simulink model "Smart_City_Communication_Infrastructure"  (R2024b)
settings: Solver=ode1  StartTime=0.0  StopTime=inf  FixedStep=Controller_Sample_Time  RelTol=1e-3  EnableMultiTasking=on
undefined symbols (not defined in the file or in its folder): DiscIntNeverNeededParam, qc_get_step_size
libraries: quarc_library x26, simulink x2
settings Model: SimulationMode=external  ExtModeTrigDuration=10000  Creator=PK  LastModifiedBy=user
settings SolverCC: AlgebraicLoopSolver=TrustRegion  PositivePriorityOrder=on
settings DataIOCC: ReturnWorkspaceOutputs=off
settings DebuggingCC: UnconnectedInputMsg=warning  UnconnectedOutputMsg=warning  UnconnectedLineMsg=warning  ArithmeticOperatorsInVariantConditions=warning
settings ModelReferenceCC: EnableRefExpFcnMdlSchedulingChecks=on
settings SFSimCC: SimUseLocalCustomCode=off  CustomCodeUndefinedFunction=UseInterfaceOnly
settings RTWCC: Description=QUARC Win64 Target Using Toolchain  SystemTargetFile=quarc_win64.tlc  TemplateMakefile=quarc_default_tmf  RTWUseLocalCustomCode=off  Toolchain=QUARC win64 | nmake (64-bit Windows)  BuildConfiguration=Faster Runs  GPUComputeCapability=3.5
settings CodeAppCC: StateflowObjectComments=on
settings STFCustomTargetCC: TargetLangStandard=C99 (ISO)  ConcurrentExecutionCompliant=on  GRTInterface=on  UseToolchainInfoCompliant=on  SystemTargetFile=quarc_win64.tlc
settings GRTTargetCC: ParMdlRefBuildCompliant=off  CompOptLevelCompliant=off  CombineOutputUpdateFcns=off  MatFileLogging=off  CPPClassGenCompliant=off  GRTInterface=on  ExtMode=on  ExtModeMexFile=quarc_comm
settings ConfigComp: CovMetricSettings=dswe

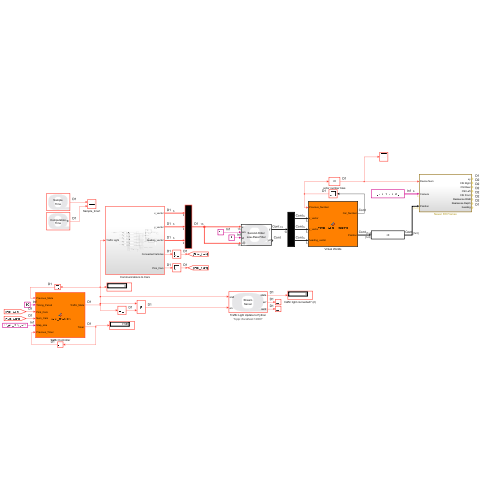
[thumbnail: Simulink's stored preview of the top-level diagram]
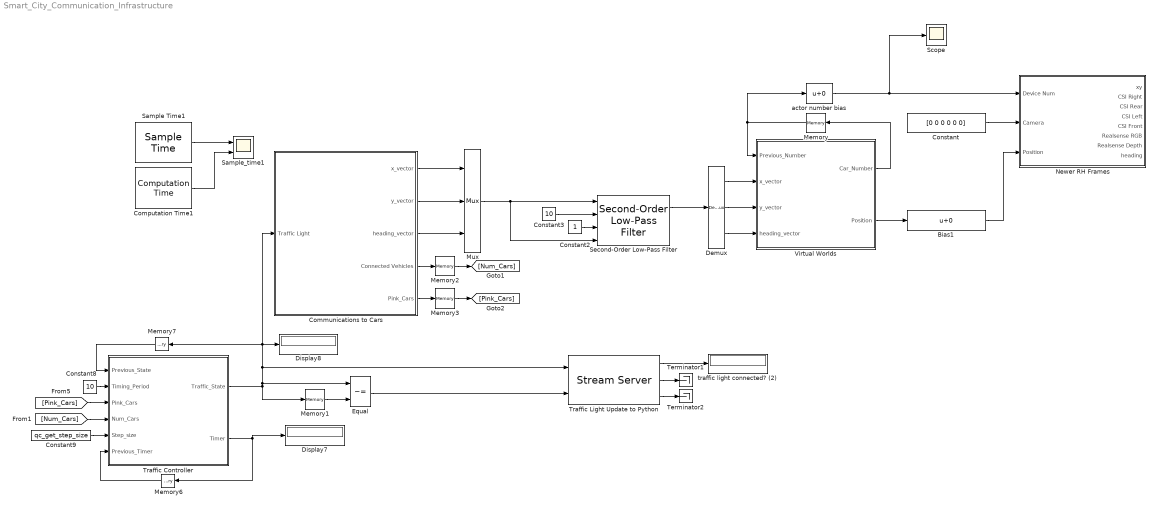
== system Smart_City_Communication_Infrastructure ==
  Bias1 : Bias  SaturateOnIntegerOverflow=off
  Communications to Cars : Subsystem
  Computation Time1 : quarc_library/Sources/Time/Computation Time  sample_time=qc_get_step_size  use_model=on  use_cpu_time=off
  Constant : Constant  Value=[0 0 0 0 0 0]
  Constant2 : Constant
  Constant3 : Constant  Value=10
  Constant8 : Constant  Value=10
  Constant9 : Constant  Value=qc_get_step_size
  Demux : Demux  Outputs=3
  Display7 : Display
  Display8 : Display
  Equal : RelationalOperator  Operator=~=  OutDataTypeStr=boolean  RndMeth=Simplest  InputSameDT=off
  Memory : Memory  InitialCondition=1  InheritSampleTime=on  LinearizeMemory=on  LinearizeAsDelay=on
  Memory1 : Memory
  Memory2 : Memory  InheritSampleTime=on  LinearizeMemory=on  LinearizeAsDelay=on
  Memory3 : Memory  InheritSampleTime=on  LinearizeMemory=on  LinearizeAsDelay=on
  Memory6 : Memory  InheritSampleTime=on  LinearizeMemory=on  LinearizeAsDelay=on
  Memory7 : Memory  InitialCondition=1  InheritSampleTime=on  LinearizeMemory=on  LinearizeAsDelay=on
  Mux : Mux  Inputs=3
  Newer RH Frames : Subsystem
  Sample Time1 : quarc_library/Sources/Time/Sample Time  Priority=-99  sample_time=qc_get_step_size
  Sample_time1 : Scope  NumInputPorts=2
  Scope : Scope
  Second-Order Low-Pass Filter : quarc_library/Continuous/Second-Order Low-Pass Filter  params_source=External (input ports)  input_width=1  input_zeta=1  input_init=0
  Terminator1 : Terminator
  Terminator2 : Terminator
  Traffic Controller : MATLAB Function  TreatAsAtomicUnit=on
  Traffic Light Update to Python : quarc_library/Communications/Basic/Stream Server  uri_source=Specify via dialog (do not evaluate)  uri=tcpip://localhost:12000  send_buffer_size=1460  receive_buffer_size=1460  byte_order=little endian (Intel - LSB first)  optimization=Minimum latency  send_options=Send most recent data  receive_options=Do not receive data  default_value=[5 5]  sample_time=-1  active=off  implementation=Use blocking I/O in a separate thread  send_fifo_size=1000  receive_fifo_size=1000  send_priority=0  receive_priority=0  send_dimensions=off  receive_dimensions=off  max_dimensions=-1  data_type=Inherited via back propagation  type_expr=BusObject
      settings: AttributesFormatString="\"tcpip://localhost:12000\""
  Virtual Worlds : MATLAB Function  TreatAsAtomicUnit=on
  actor number bias : Bias  SaturateOnIntegerOverflow=off
  traffic light connected? (2) : Display
  wires:
  Memory3/1 -> [Pink_Cars]
  Memory2/1 -> [Num_Cars]
  Memory1/1 -> Equal/2
  Constant3/1 -> Second-Order Low-Pass Filter/2
  Communications to Cars/4(Connected Vehicles) -> Memory2/1
  [Pink_Cars] -> Traffic Controller/3(Pink_Cars)
  [Num_Cars] -> Traffic Controller/4(Num_Cars)
  Second-Order Low-Pass Filter/1 -> Demux/1
  actor number bias/1 -> Scope/1, Newer RH Frames/1(Device Num)
  Constant2/1 -> Second-Order Low-Pass Filter/3
  Communications to Cars/3(heading_vector) -> Mux/3
  Virtual Worlds/1(Car_Number) -> Memory/1
  Communications to Cars/5(Pink_Cars) -> Memory3/1
  Memory6/1 -> Traffic Controller/6(Previous_Timer)
  Virtual Worlds/2(Position) -> Bias1/1
  Demux/2 -> Virtual Worlds/3(y_vector)
  Demux/1 -> Virtual Worlds/2(x_vector)
  Equal/1 -> Traffic Light Update to Python/2
  Communications to Cars/2(y_vector) -> Mux/2
  Demux/3 -> Virtual Worlds/4(heading_vector)
  Memory/1 -> actor number bias/1, Virtual Worlds/1(Previous_Number)
  Constant/1 -> Newer RH Frames/2(Camera)
  Constant8/1 -> Traffic Controller/2(Timing_Period)
  Mux/1 -> Second-Order Low-Pass Filter/1, Second-Order Low-Pass Filter/4
  Computation Time1/1 -> Sample_time1/2
  Sample Time1/1 -> Sample_time1/1
  Traffic Controller/1(Traffic_State) -> Display8/1, Communications to Cars/1(Traffic Light), Memory7/1, Traffic Light Update to Python/1, Equal/1, Memory1/1
  Communications to Cars/1(x_vector) -> Mux/1
  Traffic Controller/2(Timer) -> Display7/1, Memory6/1
  Constant9/1 -> Traffic Controller/5(Step_size)
  Memory7/1 -> Traffic Controller/1(Previous_State)
  Bias1/1 -> Newer RH Frames/3(Position)
  Traffic Light Update to Python/1 -> traffic light connected? (2)/1
  Traffic Light Update to Python/2 -> Terminator1/1
  Traffic Light Update to Python/3 -> Terminator2/1

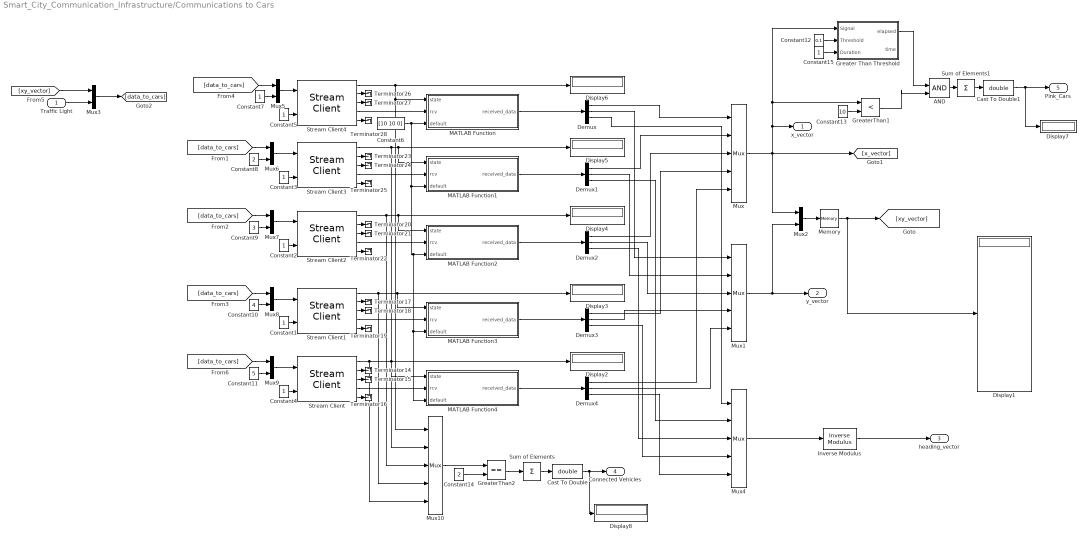
== system Smart_City_Communication_Infrastructure/Communications to Cars ==
  Traffic Light : Inport
  AND : Logic  IconShape=distinctive  AllPortsSameDT=off  OutDataTypeStr=boolean
  Cast To Double : DataTypeConversion  OutDataTypeStr=double  SaturateOnIntegerOverflow=off  RndMeth=Floor
  Cast To Double1 : DataTypeConversion  OutDataTypeStr=double  SaturateOnIntegerOverflow=off  RndMeth=Floor
  Constant{1..5,7,15} (7 alike) : Constant
  Constant10 : Constant  Value=4
  Constant11 : Constant  Value=5
  Constant12 : Constant  Value=0.1
  Constant13 : Constant  Value=10
  Constant14 : Constant  Value=2
  Constant6 : Constant  Value=[10 10 0]
  Constant8 : Constant  Value=2
  Constant9 : Constant  Value=3
  Demux{,1..4} (5 alike) : Demux  Outputs=3
  Display{1..8} (8 alike) : Display
      settings: Decimation=100
  Greater Than Threshold : Subsystem
  GreaterThan1 : RelationalOperator  Operator=<  OutDataTypeStr=boolean  RndMeth=Simplest  InputSameDT=off
  GreaterThan2 : RelationalOperator  Operator===  OutDataTypeStr=boolean  RndMeth=Simplest  InputSameDT=off
  Inverse Modulus : quarc_library/Discontinuities/Inverse Modulus  modulus=2*pi  output_derivative=off  output_revolutions=off  max_x=Inf  min_x=-Inf
  MATLAB Function : MATLAB Function  TreatAsAtomicUnit=on
  MATLAB Function1 : MATLAB Function  TreatAsAtomicUnit=on
  MATLAB Function2 : MATLAB Function  TreatAsAtomicUnit=on
  MATLAB Function3 : MATLAB Function  TreatAsAtomicUnit=on
  MATLAB Function4 : MATLAB Function  TreatAsAtomicUnit=on
  Memory : Memory  InitialCondition=10*ones(1,10)  InheritSampleTime=on  LinearizeMemory=on  LinearizeAsDelay=on
  Mux{,1,4,10} (4 alike) : Mux  Inputs=5
  Mux{2..3,5..9} (7 alike) : Mux  Inputs=2
  Stream Client : quarc_library/Communications/Basic/Stream Client  uri_source=Specify via dialog (do not evaluate)  uri=tcpip://localhost:5555?nagle='off'  send_buffer_size=1460  receive_buffer_size=1460  byte_order=little endian (Intel - LSB first)  optimization=Minimum latency  send_options=Send most recent data  receive_options=Receive most recent data  default_value=[10 10 0]  sample_time=qc_get_step_size  active=off  implementation=Use blocking I/O in a separate thread  send_fifo_size=1  receive_fifo_size=1  send_priority=0  receive_priority=0  send_dimensions=off  receive_dimensions=off  max_dimensions=-1  data_type=Inherited via back propagation  type_expr=BusObject
      settings: AttributesFormatString="\"tcpip://localhost:5555?nagle='off'\""
  Stream Client1 : quarc_library/Communications/Basic/Stream Client  uri_source=Specify via dialog (do not evaluate)  uri=tcpip://localhost:4444?nagle='off'  send_buffer_size=1460  receive_buffer_size=1460  byte_order=little endian (Intel - LSB first)  optimization=Minimum latency  send_options=Send most recent data  receive_options=Receive most recent data  default_value=[10 10 0]  sample_time=qc_get_step_size  active=off  implementation=Use blocking I/O in a separate thread  send_fifo_size=1  receive_fifo_size=1  send_priority=0  receive_priority=0  send_dimensions=off  receive_dimensions=off  max_dimensions=-1  data_type=Inherited via back propagation  type_expr=BusObject
      settings: AttributesFormatString="\"tcpip://localhost:4444?nagle='off'\""
  Stream Client2 : quarc_library/Communications/Basic/Stream Client  uri_source=Specify via dialog (do not evaluate)  uri=tcpip://192.168.2.13:1111?nagle='off'  send_buffer_size=1460  receive_buffer_size=1460  byte_order=little endian (Intel - LSB first)  optimization=Minimum latency  send_options=Send most recent data  receive_options=Receive most recent data  default_value=[10 10 0]  sample_time=qc_get_step_size  active=off  implementation=Use blocking I/O in a separate thread  send_fifo_size=1  receive_fifo_size=1  send_priority=0  receive_priority=0  send_dimensions=off  receive_dimensions=off  max_dimensions=-1  data_type=Inherited via back propagation  type_expr=BusObject
      settings: AttributesFormatString="\"tcpip://192.168.2.13:1111?nagle='off'\""
  Stream Client3 : quarc_library/Communications/Basic/Stream Client  uri_source=Specify via dialog (do not evaluate)  uri=tcpip://192.168.2.12:1111?nagle='off'  send_buffer_size=1460  receive_buffer_size=1460  byte_order=little endian (Intel - LSB first)  optimization=Minimum latency  send_options=Send most recent data  receive_options=Receive most recent data  default_value=[10 10 0]  sample_time=qc_get_step_size  active=off  implementation=Use blocking I/O in a separate thread  send_fifo_size=1  receive_fifo_size=1  send_priority=0  receive_priority=0  send_dimensions=off  receive_dimensions=off  max_dimensions=-1  data_type=Inherited via back propagation  type_expr=BusObject
      settings: AttributesFormatString="\"tcpip://192.168.2.12:1111?nagle='off'\""
  Stream Client4 : quarc_library/Communications/Basic/Stream Client  uri_source=Specify via dialog (do not evaluate)  uri=tcpip://192.168.2.11:1111?nagle='off'  send_buffer_size=1460  receive_buffer_size=1460  byte_order=little endian (Intel - LSB first)  optimization=Minimum latency  send_options=Send most recent data  receive_options=Receive most recent data  default_value=[10 10 0]  sample_time=-1  active=off  implementation=Use blocking I/O in a separate thread  send_fifo_size=1  receive_fifo_size=1  send_priority=0  receive_priority=0  send_dimensions=off  receive_dimensions=off  max_dimensions=-1  data_type=Inherited via back propagation  type_expr=BusObject
      settings: AttributesFormatString="\"tcpip://192.168.2.11:1111?nagle='off'\""
  Sum of Elements : Sum  Inputs=+
  Sum of Elements1 : Sum  Inputs=+
  Terminator{14..28} (15 alike) : Terminator
  x_vector : Outport
  y_vector : Outport  Port=2
  heading_vector : Outport  Port=3
  Connected Vehicles : Outport  Port=4
  Pink_Cars : Outport  Port=5
  wires:
  Demux4/1 -> Mux/5
  Demux1/1 -> Mux/2
  Demux/1 -> Mux/1
  Stream Client1/5 -> Terminator19/1
  Stream Client4/1 -> MATLAB Function/1(state), Mux10/1, Display6/1
  Stream Client2/3 -> Terminator21/1
  Stream Client2/2 -> Terminator20/1
  Stream Client1/3 -> Terminator18/1
  MATLAB Function4/1(received_data) -> Demux4/1
  Stream Client3/3 -> Terminator24/1
  Demux2/1 -> Mux/3
  Stream Client1/2 -> Terminator17/1
  Memory/1 -> Display1/1, [xy_vector]
  Constant4/1 -> Stream Client/2
  Stream Client4/5 -> Terminator28/1
  Stream Client/1 -> MATLAB Function4/1(state), Display2/1, Mux10/5
  Stream Client3/1 -> Mux10/2, MATLAB Function1/1(state), Display5/1
  Constant3/1 -> Stream Client3/2
  Stream Client1/1 -> Mux10/4, MATLAB Function3/1(state), Display3/1
  Constant5/1 -> Stream Client4/2
  MATLAB Function/1(received_data) -> Demux/1
  Mux/1 -> Greater Than Threshold/1(Signal), GreaterThan1/1, x_vector/1, Mux2/1, [x_vector]
  Stream Client4/2 -> Terminator26/1
  Mux1/1 -> y_vector/1, Mux2/2
  Mux2/1 -> Memory/1
  Constant6/1 -> MATLAB Function4/3(default), MATLAB Function3/3(default), MATLAB Function2/3(default), MATLAB Function1/3(default), MATLAB Function/3(default)
  Stream Client2/1 -> Mux10/3, MATLAB Function2/1(state), Display4/1
  MATLAB Function3/1(received_data) -> Demux3/1
  Stream Client/4 -> MATLAB Function4/2(rcv)
  MATLAB Function1/1(received_data) -> Demux1/1
  Demux/2 -> Mux1/1
  Constant2/1 -> Stream Client2/2
  Stream Client2/5 -> Terminator22/1
  MATLAB Function2/1(received_data) -> Demux2/1
  Demux1/2 -> Mux1/2
  Demux3/1 -> Mux/4
  Stream Client3/2 -> Terminator23/1
  Demux2/2 -> Mux1/3
  Stream Client3/4 -> MATLAB Function1/2(rcv)
  Constant1/1 -> Stream Client1/2
  Stream Client2/4 -> MATLAB Function2/2(rcv)
  Stream Client/5 -> Terminator16/1
  Stream Client1/4 -> MATLAB Function3/2(rcv)
  Stream Client4/4 -> MATLAB Function/2(rcv)
  Demux3/2 -> Mux1/4
  Stream Client/2 -> Terminator14/1
  Stream Client/3 -> Terminator15/1
  Stream Client4/3 -> Terminator27/1
  Stream Client3/5 -> Terminator25/1
  [xy_vector] -> Mux3/1
  Mux3/1 -> [data_to_cars]
  Traffic Light/1 -> Mux3/2
  Demux4/2 -> Mux1/5
  Demux4/3 -> Mux4/5
  Demux3/3 -> Mux4/4
  Demux2/3 -> Mux4/3
  Demux1/3 -> Mux4/2
  Demux/3 -> Mux4/1
  Mux4/1 -> Inverse Modulus/1
  Inverse Modulus/1 -> heading_vector/1
  Mux5/1 -> Stream Client4/1
  [data_to_cars] -> Mux5/1
  Constant7/1 -> Mux5/2
  Constant8/1 -> Mux6/2
  [data_to_cars] -> Mux6/1
  [data_to_cars] -> Mux7/1
  Constant9/1 -> Mux7/2
  Constant10/1 -> Mux8/2
  [data_to_cars] -> Mux8/1
  [data_to_cars] -> Mux9/1
  Constant11/1 -> Mux9/2
  Mux6/1 -> Stream Client3/1
  Mux7/1 -> Stream Client2/1
  Mux8/1 -> Stream Client1/1
  Mux9/1 -> Stream Client/1
  AND/1 -> Sum of Elements1/1
  Constant13/1 -> GreaterThan1/2
  GreaterThan1/1 -> AND/2
  Sum of Elements1/1 -> Cast To Double1/1
  Mux10/1 -> GreaterThan2/1
  GreaterThan2/1 -> Sum of Elements/1
  Sum of Elements/1 -> Cast To Double/1
  Constant14/1 -> GreaterThan2/2
  Cast To Double/1 -> Display8/1, Connected Vehicles/1
  Cast To Double1/1 -> Display7/1, Pink_Cars/1
  Greater Than Threshold/1(elapsed) -> AND/1
  Constant12/1 -> Greater Than Threshold/2(Threshold)
  Constant15/1 -> Greater Than Threshold/3(Duration)

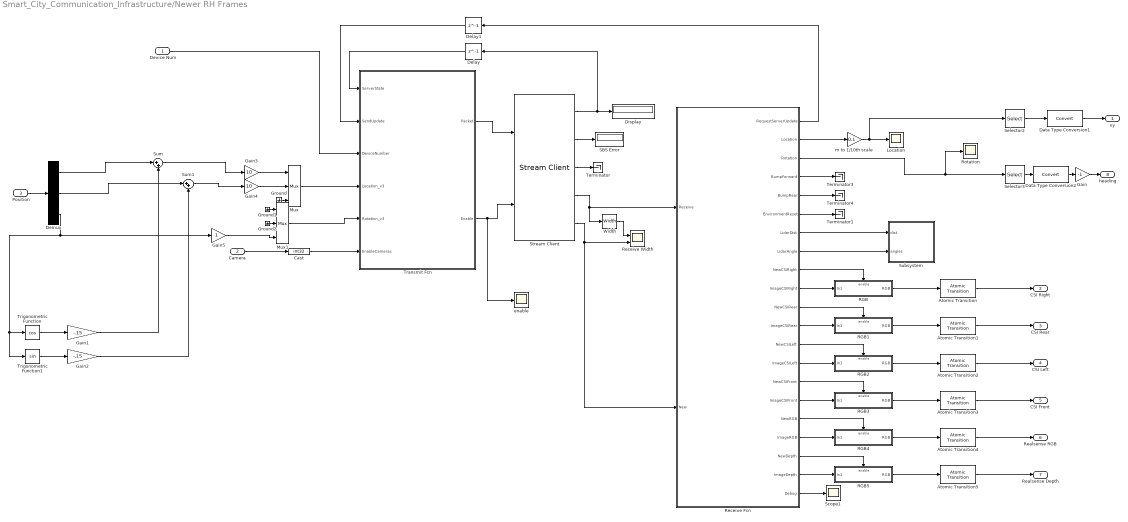
== system Smart_City_Communication_Infrastructure/Newer RH Frames ==
  Device Num : Inport
  Camera : Inport  Port=2
  Position : Inport  Port=3
  Atomic Transition{,1..5} (6 alike) : quarc_library/Advanced/Asynchronous/Atomic Transition  sample_time=cameraStepSize  data_type=Inherit: Same as input
      settings: SourceProductName=QUARC Targets
  Cast : DataTypeConversion  OutDataTypeStr=int32  SaturateOnIntegerOverflow=off  RndMeth=Floor
  Data Type Conversion1 : DataTypeConversion  SaturateOnIntegerOverflow=off  RndMeth=Floor
  Data Type Conversion2 : DataTypeConversion  SaturateOnIntegerOverflow=off  RndMeth=Floor
  Delay : Delay  DelayLength=1
  Delay1 : Delay  DelayLength=1
  Demux : Demux  Outputs=3
  Display : Display
  Gain : Gain  Gain=-1
  Gain1 : Gain  Gain=-.15
  Gain2 : Gain  Gain=-.15
  Gain3 : Gain  Gain=10
  Gain4 : Gain  Gain=10
  Gain5 : Gain
  Ground : Ground
  Ground1 : Ground
  Ground2 : Ground
  Location : Scope
  Mux : Mux  Inputs=3
  Mux1 : Mux  Inputs=3
  RGB : Subsystem
  RGB1 : Subsystem
  RGB2 : Subsystem
  RGB3 : Subsystem
  RGB4 : Subsystem
  RGB5 : Subsystem
  Receive Fcn : MATLAB Function  TreatAsAtomicUnit=on
  Receive Width : Scope  NumInputPorts=2
  Rotation : Scope
  SBS Error : Display
  Scope1 : Scope
  Selector2 : Selector  InputPortWidth=3  IndexOptions=Index vector (dialog)  Indices=1:2  OutputSizes=1
  Selector3 : Selector  InputPortWidth=3  IndexOptions=Index vector (dialog)  Indices=3  OutputSizes=1
  Stream Client : quarc_library/Communications/Basic/Stream Client  uri_source=Specify via dialog (do not evaluate)  uri=tcpip://localhost:18000?nagle='off'  send_buffer_size=100000  receive_buffer_size=800000  byte_order=little endian (Intel - LSB first)  optimization=Minimum latency  send_options=Send all data  receive_options=Receive all data  default_value=[0]  sample_time=qc_get_step_size  active=on  implementation=Use blocking I/O in a separate thread  send_fifo_size=2  receive_fifo_size=2  send_priority=0  receive_priority=0  send_dimensions=on  receive_dimensions=on  max_dimensions=800000  data_type=uint8  type_expr=BusObject
      settings: AttributesFormatString="\"tcpip://localhost:18000?nagle='off'\""
  Subsystem : Subsystem
  Sum : Sum  Inputs=|++
  Sum1 : Sum  Inputs=|++
  Terminator{,1,3..4} (4 alike) : Terminator
  Transmit Fcn : MATLAB Function  TreatAsAtomicUnit=on
  Trigonometric Function : Trigonometry  Operator=cos
  Trigonometric Function1 : Trigonometry
  Width : Width
  enable : Scope
  m to 1/10th scale : Gain  Gain=0.1
  xy : Outport
  CSI Right : Outport  Port=2
  CSI Rear : Outport  Port=3
  CSI Left : Outport  Port=4
  CSI Front : Outport  Port=5
  Realsense RGB : Outport  Port=6
  Realsense Depth : Outport  Port=7
  heading : Outport  Port=8
  wires:
  Device Num/1 -> Transmit Fcn/3(DeviceNumber)
  Transmit Fcn/2(Enable) -> enable/1, Stream Client/2
  Atomic Transition4/1 -> Realsense RGB/1
  Receive Fcn/10(ImageCSIRight) -> RGB/1(In1)
  RGB5/1(RGB) -> Atomic Transition5/1
  Width/1 -> Receive Width/1
  Receive Fcn/17(NewRGB) -> RGB4/Enable
  RGB3/1(RGB) -> Atomic Transition3/1
  Receive Fcn/13(NewCSILeft) -> RGB2/Enable
  Receive Fcn/12(ImageCSIRear) -> RGB1/1(In1)
  Receive Fcn/16(ImageCSIFront) -> RGB3/1(In1)
  Receive Fcn/9(NewCSIRight) -> RGB/Enable
  Receive Fcn/8(LidarAngle) -> Subsystem/2(angles)
  Receive Fcn/5(BumpRear) -> Terminator4/1
  RGB1/1(RGB) -> Atomic Transition1/1
  Atomic Transition5/1 -> Realsense Depth/1
  RGB4/1(RGB) -> Atomic Transition4/1
  Receive Fcn/1(RequestServerUpdate) -> Delay1/1
  Stream Client/2 -> SBS Error/1
  Atomic Transition2/1 -> CSI Left/1
  Receive Fcn/7(LidarDist) -> Subsystem/1(dist)
  Receive Fcn/20(ImageDepth) -> RGB5/1(In1)
  Receive Fcn/21(Debug) -> Scope1/1
  Receive Fcn/18(ImageRGB) -> RGB4/1(In1)
  RGB2/1(RGB) -> Atomic Transition2/1
  Atomic Transition3/1 -> CSI Front/1
  Stream Client/1 -> Display/1, Delay/1
  Stream Client/5 -> Receive Fcn/2(New), Receive Width/2
  Receive Fcn/15(NewCSIFront) -> RGB3/Enable
  Receive Fcn/19(NewDepth) -> RGB5/Enable
  Receive Fcn/14(ImageCSILeft) -> RGB2/1(In1)
  Delay/1 -> Transmit Fcn/1(ServerState)
  Receive Fcn/11(NewCSIRear) -> RGB1/Enable
  m to 1/10th scale/1 -> Selector2/1, Location/1
  RGB/1(RGB) -> Atomic Transition/1
  Atomic Transition1/1 -> CSI Rear/1
  Delay1/1 -> Transmit Fcn/2(SendUpdate)
  Receive Fcn/4(BumpForward) -> Terminator3/1
  Transmit Fcn/1(Packet) -> Stream Client/1
  Stream Client/4 -> Width/1, Receive Fcn/1(Receive)
  Stream Client/3 -> Terminator/1
  Camera/1 -> Cast/1
  Receive Fcn/6(EnvironmentReset) -> Terminator1/1
  Cast/1 -> Transmit Fcn/6(EnableCameras)
  Atomic Transition/1 -> CSI Right/1
  Data Type Conversion1/1 -> xy/1
  Selector2/1 -> Data Type Conversion1/1
  Gain/1 -> heading/1
  Selector3/1 -> Data Type Conversion2/1
  Data Type Conversion2/1 -> Gain/1
  Mux/1 -> Transmit Fcn/4(Location_v3)
  Mux1/1 -> Transmit Fcn/5(Rotation_v3)
  Position/1 -> Demux/1
  Demux/3 -> Gain5/1, Trigonometric Function1/1, Trigonometric Function/1
  Trigonometric Function/1 -> Gain1/1
  Trigonometric Function1/1 -> Gain2/1
  Demux/1 -> Sum/1
  Gain1/1 -> Sum/2
  Sum/1 -> Gain3/1
  Gain3/1 -> Mux/1
  Gain4/1 -> Mux/2
  Sum1/1 -> Gain4/1
  Demux/2 -> Sum1/1
  Gain2/1 -> Sum1/2
  Gain5/1 -> Mux1/3
  Receive Fcn/2(Location) -> m to 1/10th scale/1
  Receive Fcn/3(Rotation) -> Rotation/1, Selector3/1
  Ground/1 -> Mux/3
  Ground1/1 -> Mux1/1
  Ground2/1 -> Mux1/2

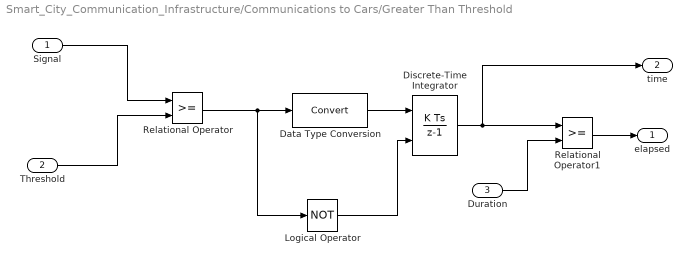
== system Smart_City_Communication_Infrastructure/Communications to Cars/Greater Than Threshold ==
  Signal : Inport
  Threshold : Inport  Port=2
  Duration : Inport  Port=3
  Data Type Conversion : DataTypeConversion  SaturateOnIntegerOverflow=off  RndMeth=Floor
  Discrete-Time Integrator : DiscreteIntegrator  Priority=1  ExternalReset=level  SampleTime=qc_get_step_size  ICPrevOutput=DiscIntNeverNeededParam  ICPrevScaledInput=DiscIntNeverNeededParam
  Logical Operator : Logic  Operator=NOT  AllPortsSameDT=off  OutDataTypeStr=boolean
  Relational Operator : RelationalOperator  InputSameDT=off
  Relational Operator1 : RelationalOperator  InputSameDT=off
  elapsed : Outport  VectorParamsAs1DForOutWhenUnconnected=off
  time : Outport  Port=2  VectorParamsAs1DForOutWhenUnconnected=off
  wires:
  Data Type Conversion/1 -> Discrete-Time Integrator/1
  Signal/1 -> Relational Operator/1
  Threshold/1 -> Relational Operator/2
  Relational Operator/1 -> Data Type Conversion/1, Logical Operator/1
  Logical Operator/1 -> Discrete-Time Integrator/2
  Discrete-Time Integrator/1 -> Relational Operator1/1, time/1
  Duration/1 -> Relational Operator1/2
  Relational Operator1/1 -> elapsed/1

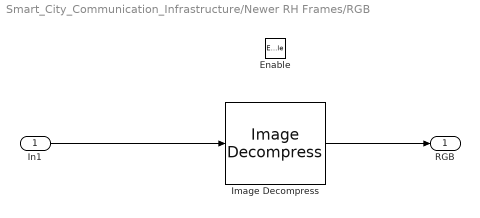
== system Smart_City_Communication_Infrastructure/Newer RH Frames/RGB ==
  In1 : Inport
  Enable : EnablePort  StatesWhenEnabling=reset
  Image Decompress : quarc_library/Image Processing/Generic/Image Decompress  algorithm=JPEG  resolution=custom  width=820  height=410  output_format=MATLAB RGB (HxWx3)  data_type=uint8
      settings: AttributesFormatString=(%<algorithm>)  SourceProductName=QUARC Targets
  RGB : Outport  VectorParamsAs1DForOutWhenUnconnected=off
  wires:
  In1/1 -> Image Decompress/1
  Image Decompress/1 -> RGB/1

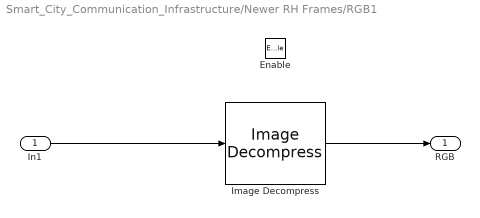
== system Smart_City_Communication_Infrastructure/Newer RH Frames/RGB1 ==
  In1 : Inport
  Enable : EnablePort  StatesWhenEnabling=reset
  Image Decompress : quarc_library/Image Processing/Generic/Image Decompress  algorithm=JPEG  resolution=custom  width=820  height=410  output_format=MATLAB RGB (HxWx3)  data_type=uint8
      settings: AttributesFormatString=(%<algorithm>)  SourceProductName=QUARC Targets
  RGB : Outport  VectorParamsAs1DForOutWhenUnconnected=off
  wires:
  In1/1 -> Image Decompress/1
  Image Decompress/1 -> RGB/1

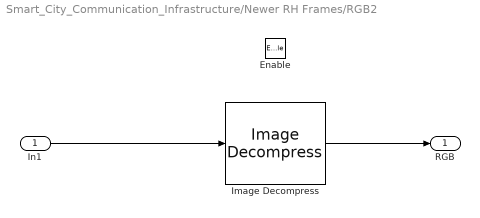
== system Smart_City_Communication_Infrastructure/Newer RH Frames/RGB2 ==
  In1 : Inport
  Enable : EnablePort  StatesWhenEnabling=reset
  Image Decompress : quarc_library/Image Processing/Generic/Image Decompress  algorithm=JPEG  resolution=custom  width=820  height=410  output_format=MATLAB RGB (HxWx3)  data_type=uint8
      settings: AttributesFormatString=(%<algorithm>)  SourceProductName=QUARC Targets
  RGB : Outport  VectorParamsAs1DForOutWhenUnconnected=off
  wires:
  In1/1 -> Image Decompress/1
  Image Decompress/1 -> RGB/1

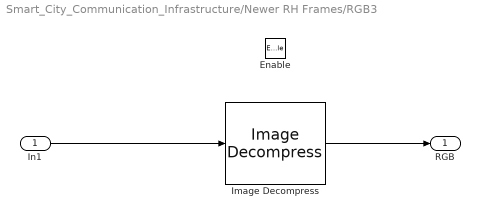
== system Smart_City_Communication_Infrastructure/Newer RH Frames/RGB3 ==
  In1 : Inport
  Enable : EnablePort  StatesWhenEnabling=reset
  Image Decompress : quarc_library/Image Processing/Generic/Image Decompress  algorithm=JPEG  resolution=custom  width=820  height=410  output_format=MATLAB RGB (HxWx3)  data_type=uint8
      settings: AttributesFormatString=(%<algorithm>)  SourceProductName=QUARC Targets
  RGB : Outport  VectorParamsAs1DForOutWhenUnconnected=off
  wires:
  In1/1 -> Image Decompress/1
  Image Decompress/1 -> RGB/1

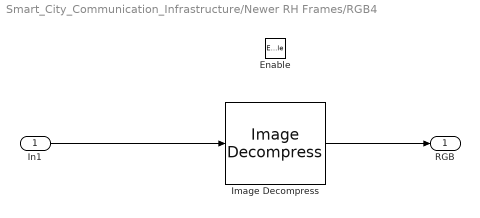
== system Smart_City_Communication_Infrastructure/Newer RH Frames/RGB4 ==
  In1 : Inport
  Enable : EnablePort  StatesWhenEnabling=reset
  Image Decompress : quarc_library/Image Processing/Generic/Image Decompress  algorithm=JPEG  resolution=640 x 480  width=640  height=480  output_format=MATLAB RGB (HxWx3)  data_type=uint8
      settings: AttributesFormatString=(%<algorithm>)  SourceProductName=QUARC Targets
  RGB : Outport  VectorParamsAs1DForOutWhenUnconnected=off
  wires:
  In1/1 -> Image Decompress/1
  Image Decompress/1 -> RGB/1

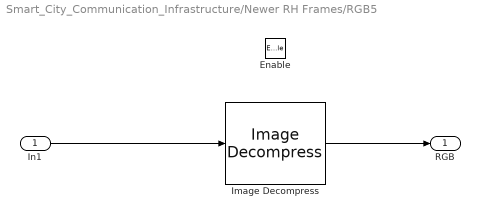
== system Smart_City_Communication_Infrastructure/Newer RH Frames/RGB5 ==
  In1 : Inport
  Enable : EnablePort  StatesWhenEnabling=reset
  Image Decompress : quarc_library/Image Processing/Generic/Image Decompress  algorithm=JPEG  resolution=640 x 480  width=640  height=480  output_format=MATLAB RGB (HxWx3)  data_type=uint8
      settings: AttributesFormatString=(%<algorithm>)  SourceProductName=QUARC Targets
  RGB : Outport  VectorParamsAs1DForOutWhenUnconnected=off
  wires:
  In1/1 -> Image Decompress/1
  Image Decompress/1 -> RGB/1

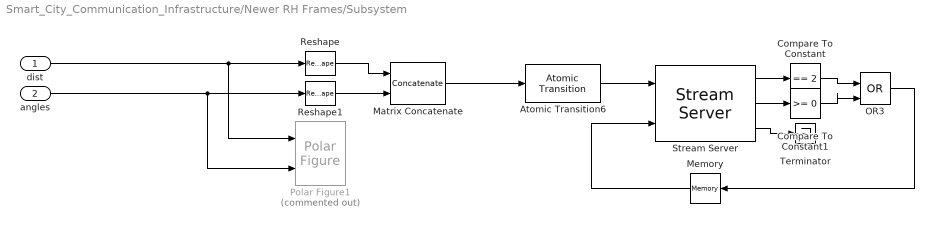
== system Smart_City_Communication_Infrastructure/Newer RH Frames/Subsystem ==
  dist : Inport
  angles : Inport  Port=2
  Atomic Transition6 : quarc_library/Advanced/Asynchronous/Atomic Transition  sample_time=cameraStepSize  data_type=Inherit: Same as input
      settings: SourceProductName=QUARC Targets
  Compare To Constant : simulink/Logic and Bit Operations/Compare To Constant  relop===  const=2  OutDataTypeStr=boolean
  Compare To Constant1 : simulink/Logic and Bit Operations/Compare To Constant  relop=>=  const=0  OutDataTypeStr=boolean
  Matrix Concatenate : Concatenate  Mode=Multidimensional array  ConcatenateDimension=3
  Memory : Memory  InheritSampleTime=on
  OR3 : Logic  Operator=OR  IconShape=distinctive  AllPortsSameDT=off  OutDataTypeStr=boolean
  Polar Figure1 : quarc_library/Sinks/Figures/Polar Figure  Commented=on  figure_mode=Use figure window  figure_tag=figure1  axes_tag=axes1  plot_mode=Frame-based  minimum_rho=0  maximum_rho=80  minimum_theta=0  maximum_theta=360  zero_location=top  direction=clockwise  buffer_size=1  update_rate=100  sample_time=-1  initial_position="866  198  814  692"  initial_visibility=off  line1_style=None  line1_width=0.5  line1_color=[0 0.4470 0.7410]  marker1=Circle (o)  marker1_size=1  marker1_edge_color=[0 0.447059 0.741176]  marker1_face_color=[0 0.447059 0.741176]  line2_style=Solid line (-)  line2_width=0.5  line2_color=[0.85098 0.32549 0.0980392]  marker2=None  marker2_size=6  marker2_edge_color=[0.85098 0.32549 0.0980392]  marker2_face_color=[0.85098 0.32549 0.0980392]  line3_style=Solid line (-)  line3_width=0.5  line3_color=[0.929412 0.694118 0.12549]  marker3=None  marker3_size=6  marker3_edge_color=[0.929412 0.694118 0.12549]  marker3_face_color=[0.929412 0.694118 0.12549]  line4_style=Solid line (-)  line4_width=0.5  line4_color=[0.494118 0.184314 0.556863]  marker4=None  marker4_size=6  marker4_edge_color=[0.494118 0.184314 0.556863]  marker4_face_color=[0.494118 0.184314 0.556863]  line5_style=Solid line (-)  line5_width=0.5  line5_color=[0.466667 0.67451 0.188235]  marker5=None  marker5_size=6  marker5_edge_color=[0.466667 0.67451 0.188235]  marker5_face_color=[0.466667 0.67451 0.188235]
      settings: SourceProductName=QUARC Targets
  Reshape : Reshape  OutputDimensionality=Customize  OutputDimensions=[64,64]
  Reshape1 : Reshape  OutputDimensionality=Customize  OutputDimensions=[64,64]
  Stream Server : quarc_library/Communications/Basic/Stream Server  uri_source=Specify via dialog (do not evaluate)  uri=tcpip://localhost:18966  send_buffer_size=8*4096*2  receive_buffer_size=1460  byte_order=little endian (Intel - LSB first)  optimization=Minimum latency  send_options=Send most recent data  receive_options=Do not receive data  default_value=[0]  sample_time=cameraStepSize  active=off  implementation=Use blocking I/O in a separate thread  send_fifo_size=1000  receive_fifo_size=1000  send_priority=0  receive_priority=0  send_dimensions=off  receive_dimensions=off  max_dimensions=-1  data_type=Inherited via back propagation  type_expr=BusObject
      settings: AttributesFormatString="\"tcpip://localhost:18966\""
  Terminator : Terminator
  wires:
  Stream Server/1 -> Compare To Constant/1
  Compare To Constant/1 -> OR3/1
  Atomic Transition6/1 -> Stream Server/1
  Reshape/1 -> Matrix Concatenate/1
  dist/1 -> Polar Figure1/1, Reshape/1
  Memory/1 -> Stream Server/2
  Reshape1/1 -> Matrix Concatenate/2
  OR3/1 -> Memory/1
  Stream Server/2 -> Compare To Constant1/1
  Matrix Concatenate/1 -> Atomic Transition6/1
  Compare To Constant1/1 -> OR3/2
  angles/1 -> Polar Figure1/2, Reshape1/1
  Stream Server/3 -> Terminator/1

== matlab function Smart_City_Communication_Infrastructure/Newer RH Frames/Transmit Fcn ==
  settings: updateMethod=DISCRETE  sampleTime=qc_get_step_size
  data: Packet output size=65537; ServerState input; SendUpdate input; Enable output; DeviceNumber input; Location_v3 input; Rotation_v3 input; EnableCameras input
function [Packet,Enable] = QCarApplicationWorkspaceMakePacketData(ServerState, SendUpdate, DeviceNumber, Location_v3, Rotation_v3, EnableCameras) 

% Be sure to set the maximum signal size of the variable size Packet port 
% in Simulink->Edit Data of the editor window.  Size should be 65537 or
% larger to ensure that the stream server generates a 4 byte packet size.

%% Setup
persistent LastServerState;

if isempty(LastServerState)
    LastServerState = uint8(0);
end

Enable = 0;
Packet = uint8([]);


%% Send new State Container or On connection
% Previous state processed, send a new one
if (SendUpdate) || ((ServerState == 2) && (LastServerState ~= 2))
%     Packet = QCarMakeCommandVelocityStateContainer(DeviceNumber, Forward_And_Steering, Lights);
 Packet = QCarMakeSetTransformContainer(DeviceNumber, Location_v3, Rotation_v3, 0, 0, 0, 0, 0, 0);
    
    for (index = 1:6)
        if (EnableCameras(index))
            Packet = [Packet; QCarMakeCameraRequestContainer(DeviceNumber, index-1)];
        end
    end
    %Packet = [Packet; QCarMakeLidarRequestContainer(DeviceNumber)];
end

%% Transmit
% If we have data to send, enable the transmit
PacketLength = length(Packet);

if (PacketLength > 0)
    % Add magic byte.  This is just for error handling and isn't typically
    % required in simulink, but useful in lower-level languages like Python
    Packet = [uint8(123); Packet];
    
    Enable = 1; 
end


LastServerState = ServerState;

== matlab function Smart_City_Communication_Infrastructure/Traffic Controller ==
  data: Previous_State input; Timing_Period input; Pink_Cars input; Num_Cars input; Traffic_State output; Step_size input; Previous_Timer input; Timer output
function [Traffic_State, Timer]  = Traffic_Controller (Previous_State, Timing_Period, Pink_Cars, Num_Cars, Step_size, Previous_Timer)
%#codegen
Traffic_State = Previous_State;
Timer = Previous_Timer + Step_size;

if Num_Cars == 0
    Pink_Timing = Timing_Period;
    Blue_Timing = Timing_Period;
    Blue_Cars = -1;
    Pink_Cars = -1;
else
    Blue_Cars = Num_Cars - Pink_Cars;
    Pink_Timing = Pink_Cars/Num_Cars*Timing_Period;
    Blue_Timing =Blue_Cars/Num_Cars*Timing_Period;
end

switch Traffic_State
    % Case 0 - Red Light, Case 1 - Green Light
    
    case 0
        if ((Timer > Blue_Timing) && (Blue_Cars < Num_Cars))
            Traffic_State = 1;
            Timer = 0;
        end
        
    case 1
        if ((Timer > Pink_Timing) && (Pink_Cars < Num_Cars))
            Traffic_State = 0;
            Timer = 0;
        end
        
end
end

== matlab function Smart_City_Communication_Infrastructure/Communications to Cars/MATLAB Function1 ==
  data: state input; received_data output; rcv input; default input
function received_data = state_checker (state, rcv, default)
received_data = rcv;
if state == 0
    received_data = default;
end
end

== matlab function Smart_City_Communication_Infrastructure/Communications to Cars/MATLAB Function ==
  data: state input; received_data output; rcv input; default input
function received_data = state_checker (state, rcv, default)
received_data = rcv;
if state == 0
    received_data = default;
end
end

== matlab function Smart_City_Communication_Infrastructure/Communications to Cars/MATLAB Function2 ==
  data: state input; received_data output; rcv input; default input
function received_data = state_checker (state, rcv, default)
received_data = rcv;
if state == 0
    received_data = default;
end
end

== matlab function Smart_City_Communication_Infrastructure/Communications to Cars/MATLAB Function3 ==
  data: state input; received_data output; rcv input; default input
function received_data = state_checker (state, rcv, default)
received_data = rcv;
if state == 0
    received_data = default;
end
end

== matlab function Smart_City_Communication_Infrastructure/Communications to Cars/MATLAB Function4 ==
  data: state input; received_data output; rcv input; default input
function received_data = state_checker (state, rcv, default)
received_data = rcv;
if state == 0
    received_data = default;
end
end

== matlab function Smart_City_Communication_Infrastructure/Virtual Worlds ==
  data: Previous_Number input; x_vector input; Car_Number output; y_vector input; heading_vector input; Position output
function [Car_Number, Position]  = Virtual_World_Positions (Previous_Number, x_vector, y_vector, heading_vector)
Car_Number = Previous_Number;
Position = [0 0 0];

switch Previous_Number
    
    case 1
        % Send car 1 info
        Position = [x_vector(1), y_vector(1), heading_vector(1)];
        Car_Number = 2;
        
    case 2
        % Send car 2 info
        Position = [x_vector(2), y_vector(2), heading_vector(2)];
        Car_Number = 3;
        
    case 3
        % Send car 3 info
        Position = [x_vector(3), y_vector(3), heading_vector(3)];
        Car_Number = 1;

end
end

== matlab function Smart_City_Communication_Infrastructure/Newer RH Frames/Receive Fcn ==
  data: Receive input size=800000; RequestServerUpdate output; New input; Location output; Rotation output; BumpForward output; BumpRear output; EnvironmentReset output; LidarDist output; LidarAngle output; NewCSIRight output; ImageCSIRight output size=100000; NewCSIRear output; ImageCSIRear output size=100000; NewCSILeft output; ImageCSILeft output size=100000; NewCSIFront output; ImageCSIFront output size=100000; NewRGB output; ImageRGB output size=100000; NewDepth output; ImageDepth output size=100000; Debug output
function [RequestServerUpdate, Location, Rotation, BumpForward, BumpRear, EnvironmentReset, LidarDist, LidarAngle, ...
    NewCSIRight, ImageCSIRight, ...
    NewCSIRear, ImageCSIRear, ...
    NewCSILeft, ImageCSILeft, ...
    NewCSIFront, ImageCSIFront, ...
    NewRGB, ImageRGB, ...
    NewDepth, ImageDepth, ...
    Debug]  = QCarApplicationWorkspaceDecodeDataPacket(Receive, New)

%% Setup

LIDAR_SAMPLES = 4096;
LIDAR_RANGE = 80;

persistent iLocation;
persistent iRotation;
persistent iBumpForward;
persistent iBumpRear;
persistent lastLidarDist;
persistent lastLidarAngle;

if isempty(iLocation)
    iLocation = [single(0); single(0); single(0)];
    iRotation = [single(0); single(0); single(0)];
    iBumpForward = uint8(0);
    iBumpRear = uint8(0);
    
    quarter_angle = linspace(0, 45, LIDAR_SAMPLES/8);
    lens_curve = -0.0077*quarter_angle.^2 + 1.3506*quarter_angle;
    lens_curve_rad = lens_curve/180*pi;
    
    lastLidarAngle = [-1*flip(lens_curve_rad) ...
        lens_curve_rad ...
        pi/2 - 1*flip(lens_curve_rad) ...
        pi/2 + lens_curve_rad ...
        pi - 1*flip(lens_curve_rad) ...
        pi + lens_curve_rad ...
        pi*3/2 - 1*flip(lens_curve_rad) ...
        pi*3/2 + lens_curve_rad];
    
    lastLidarDist = zeros(1,LIDAR_SAMPLES);
end

% Need to assign outputs here even though they are reassigned at the end
% since matlab can't determine the signal widths
Location = [single(0); single(0); single(0)];
Rotation = [single(0); single(0); single(0)];
BumpForward = uint8(0);
BumpRear = uint8(0);
EnvironmentReset = 0;

LidarAngle = zeros(1,LIDAR_SAMPLES);
LidarDist = zeros(1,LIDAR_SAMPLES);

ImageCSIRight = uint8([]);
NewCSIRight = 0;
ImageCSIRear = uint8([]);
NewCSIRear = 0;
ImageCSILeft = uint8([]);
NewCSILeft = 0;
ImageCSIFront = uint8([]);
NewCSIFront = 0;
ImageRGB = uint8([]);
NewRGB = 0;
ImageDepth = uint8([]);
NewDepth = 0;


RequestServerUpdate = uint8(0);
PacketSize = length(Receive);

Debug = int32(0);

% Packet > 0, new data, and magic number in first index
if ((PacketSize > 0) && (New == 1) && (Receive(1) == uint8(123)))
    
    %skip magic number
    Index = int32(2);
    
    while(Index <= PacketSize)
        
        %% Get container details
        ContainerSize = typecast(uint8(flip(Receive(Index:Index+3))), 'int32');
        DeviceID = typecast(uint8(flip(Receive(Index+4:Index+7))), 'int32');
        DeviceNum = typecast(uint8(flip(Receive(Index+8:Index+11))), 'int32');
        DeviceFunction = uint8(Receive(Index+12));
        PayloadStart = Index+13;
        PayloadEnd = Index+ContainerSize-1;
        
        %% Pass container to appropriate decoding function
        if (DeviceID == 160) %is this a QCar container?
            
            if (DeviceFunction == 11) %UE4 State Response
                [iLocation, iRotation, iBumpForward, iBumpRear] = QCarDecodeUE4VelocityStateContainer(Receive, PayloadStart);
                RequestServerUpdate = uint8(11);
            elseif (DeviceFunction == 13) %UE4 State Response
%                 [iLocation, iRotation, iBumpForward, iBumpRear] = QCarDecodeUE4VelocityStateContainer(Receive, PayloadStart);
                RequestServerUpdate = uint8(13);
                
            elseif (DeviceFunction == 101) % Pull out RGB payload for external processing
                CameraNum = typecast(uint8(flip(Receive(PayloadStart:PayloadStart+3))), 'int32');
                ImageSize = typecast(uint8(flip(Receive(PayloadStart+4:PayloadStart+7))), 'int32');
                
                if CameraNum == 0
                    ImageCSIRight = Receive(PayloadStart+8:PayloadEnd);
                    NewCSIRight = 1;
                    
                elseif CameraNum == 1
                    ImageCSIRear = Receive(PayloadStart+8:PayloadEnd);
                    NewCSIRear = 1;
                    
                elseif CameraNum == 2
                    ImageCSILeft = Receive(PayloadStart+8:PayloadEnd);
                    NewCSILeft = 1;
                    
                elseif CameraNum == 3
                    ImageCSIFront = Receive(PayloadStart+8:PayloadEnd);
                    NewCSIFront = 1;
                    
                elseif CameraNum == 4
                    ImageRGB = Receive(PayloadStart+8:PayloadEnd);
                    NewRGB = 1;
                    
                elseif CameraNum == 5
                    ImageDepth = Receive(PayloadStart+8:PayloadEnd);
                    NewDepth = 1;
                end
                RequestServerUpdate = uint8(1);
                
            elseif (DeviceFunction == 111) % Process LIDAR
                [lastLidarDist] = QCarDecodeLidarContainer(Receive, PayloadStart, LIDAR_SAMPLES, LIDAR_RANGE);
                RequestServerUpdate = uint8(1);
            end
        elseif (DeviceID == 1001) %Simulink notification
            if (DeviceFunction == 200) %Reset button
                EnvironmentReset = 1;
            end
            
            
            
        end
        
        
        %% Process next container if any data is left.
        Index = Index+ContainerSize;
    end
    
    
end

Location = iLocation;
Rotation = iRotation;
BumpForward = iBumpForward;
BumpRear = iBumpRear;
LidarDist = lastLidarDist;
LidarAngle = lastLidarAngle;
